simulink library "sm_trackV_lib_frame_idlerArm_i2u0l3"  (R2026a)
settings: Solver=VariableStepAuto
undefined symbols (not defined in the file): Trac, X, Y, Z
libraries: sm_lib x16
Description:
  | Copyright 2023-2026 The MathWorks, Inc.
settings Model: Creator=smiller  LastModifiedBy=smiller

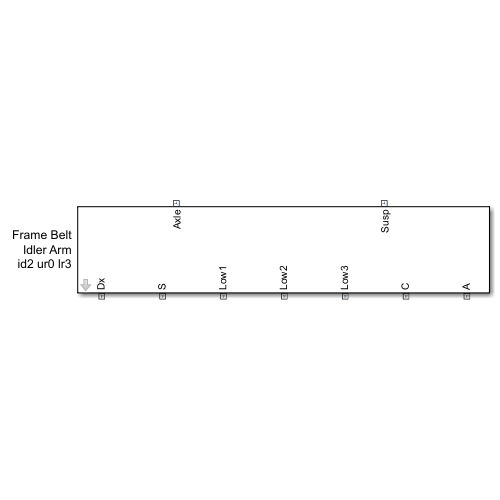
[thumbnail: Simulink's stored preview of the top-level diagram]
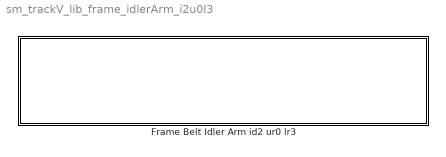
== system sm_trackV_lib_frame_idlerArm_i2u0l3 ==
  Frame Belt Idler Arm id2 ur0 lr3 : Subsystem  mask(Frame for Sprocket, Rollers (3), Fixed Idler, Idler Arm){popup_leftOrRight=Right, popup_trackFrame=Revolute, roller_lower_x=Trac.Frame.SprkOffLon.Lower, idlerArm_x=Trac.Frame.SprkOffLon.IdlerArm, idlerFix_x=Trac.Frame.SprkOffLon.IdlerR, tensionC_x=Trac.Frame.SprkOffLon.TensionC, frame_pivot_x=Trac.Frame.SprkOffLon.PivotFra, axle_x=Trac.Frame.SprkOffLon.Axle, roller_lower_y=Trac.Frame.SprkOffVer.Lower, idlerArm_y=Trac.Frame.SprkOffVer.IdlerArm, idlerFix_y=Trac.Frame.SprkOffVer.IdlerR, tensionC_y=Trac.Frame.SprkOffVer.TensionC, frame_pivot_y=Trac.Frame.SprkOffVer.PivotFra, axle_y=Trac.Frame.SprkOffVer.Axle, frame_roller_cg_offset=Trac.Frame.TrackFrame.CG, frame_roller_mass=Trac.Frame.TrackFrame.Mass, frame_roller_moi=Trac.Frame.TrackFrame.MOI, frame_roller_poi=Trac.Frame.TrackFrame.POI, frame_cg_offset=Trac.Frame.SprkFrame.CG, frame_mass=Trac.Frame.SprkFrame.Mass, frame_moi=Trac.Frame.SprkFrame.MOI, frame_poi=Trac.Frame.SprkFrame.POI, frame_susp_offset=Trac.Frame.SuspOffset, roller_frame_pivot_range=Trac.Frame.PivotFra.Range, roller_frame_pivot_k=Trac.Frame.PivotFra.LimitK, roller_frame_pivot_b=Trac.Frame.PivotFra.LimitB, roller_frame_pivot_tw=Trac.Frame.PivotFra.LimitTW}
      mask prompts: popup_leftOrRight "Left or Right"; popup_trackFrame "Track Frame"; roller_lower_x "Lower Rollers (vector) (m)"; idlerArm_x "Idler Arm (m)"; idlerFix_x "Idler Wheel Fixed (m)"; tensionC_x "Tensioner Cylinder (m)"; frame_pivot_x "Frame Pivot (m)"; axle_x "Axle (m)"; roller_lower_y "Lower Rollers (m)"; idlerArm_y "Idler Arm (m)"; idlerFix_y "Idler Wheel Fixed (m)"; tensionC_y "Tensioner Cylinder (m)"; frame_pivot_y "Frame Pivot (m)"; axle_y "Axle (m)"; frame_roller_cg_offset "CG Offset from Sprocket [x y z] (m)"; frame_roller_mass "Mass (kg)"; frame_roller_moi "Moments of Inertia [Ixx Iyy Izz] (kg*m^2)"; frame_roller_poi "Products of Inertia [Ixx Iyy Izz] (kg*m^2)"; frame_cg_offset "CG Offset from Sprocket [x y z] (m)"; frame_mass "Mass (kg)"; frame_moi "Moments of Inertia [Ixx Iyy Izz] (kg*m^2)"; frame_poi "Products of Inertia [Ixx Iyy Izz] (kg*m^2)"; frame_susp_offset "Suspension Offset from Sprocket [x y z] (m)"; roller_frame_pivot_range "Range (deg)"; roller_frame_pivot_k "Stop stiffness (N*m/deg)"; roller_frame_pivot_b "Stop damping (N*m/(deg*sec)"; roller_frame_pivot_tw "Stop transition width (deg)"
      mask help: Models frame locations for sprocket, 3 lower rollers, 1 fixed idler, 1 idler arm, and tensioner cylinder. Frame positions are all relative to sprocket center.
      mask init:
      | set_param([gcb '/Frame Connection'],'LabelModeActiveChoice',...
      |     get_param(gcb,'popup_trackFrame'))
      mask TypeOptions popup_trackFrame: Revolute | Fixed
      mask TypeOptions roller_frame_pivot_range: Frame Connection/roller_frame_pivot_range
      mask TypeOptions roller_frame_pivot_k: Frame Connection/roller_frame_pivot_k
      mask TypeOptions roller_frame_pivot_b: Frame Connection/roller_frame_pivot_b
      mask TypeOptions roller_frame_pivot_tw: Frame Connection/roller_frame_pivot_tw
      mask DialogControl cont_frame Prompt: Frame
      mask DialogControl cont_offset_x Prompt: Longitudinal Offsets from Sprocket
      mask DialogControl cont_offset_y Prompt: Vertical Offsets
      mask DialogControl cont_mass Prompt: Mass and Inertia
      mask DialogControl cont_roller_frame Prompt: Roller Frame
      mask DialogControl cont_sprk_frame Prompt: Sprocket_frame
      mask DialogControl cont_susp Prompt: Suspension Offsets
      mask DialogControl cont_framepviot Prompt: Frame Pivot (revolute only)

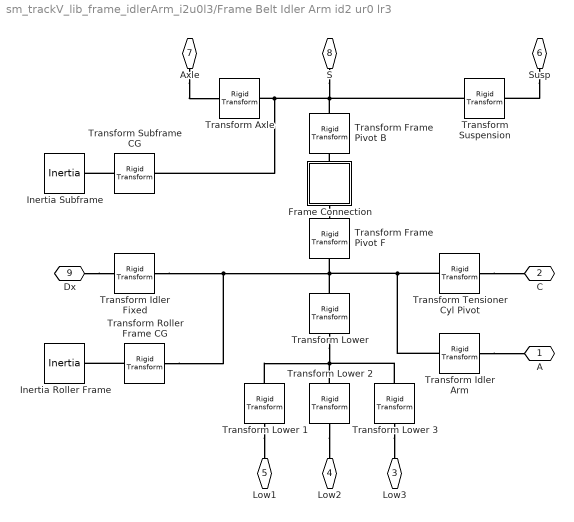
== system sm_trackV_lib_frame_idlerArm_i2u0l3/Frame Belt Idler Arm id2 ur0 lr3 ==
  Frame Connection : Subsystem  Variant=on  VariantControlMode=label  VariantControl=Revolute  LabelModeActiveChoice=Revolute  mask{roller_frame_pivot_range=roller_frame_pivot_range, roller_frame_pivot_k=roller_frame_pivot_k, roller_frame_pivot_b=roller_frame_pivot_b, roller_frame_pivot_tw=roller_frame_pivot_tw}
      mask prompts: roller_frame_pivot_range "Roller frame pivot range (deg)"; roller_frame_pivot_k "Roller frame pivot stop stiffness (N*m/deg)"; roller_frame_pivot_b "Roller frame pivot stop damping(N*m/(deg*sec)"; roller_frame_pivot_tw "Roller frame pivot stop transition width (deg)"
      settings: AttributesFormatString=%<LabelModeActiveChoice>
      mask Display: disp(' ')
  Inertia Roller Frame : sm_lib/Body Elements/Inertia  InertiaType=Custom  Mass=frame_roller_mass  MassUnits=kg  CenterOfMass=[0 0 0]  CenterOfMassUnits=m  MomentsOfInertia=frame_roller_moi  MomentsOfInertiaUnits=kg*m^2  ProductsOfInertia=frame_roller_poi  ProductsOfInertiaUnits=kg*m^2  GraphicType=None  MarkerShape=Frame  MarkerSize=20  GraphicVisPropType=SimpleVisualProperties  GraphicDiffuseColor=[0.5 0.5 0.5]  GraphicOpacity=1.0  GraphicSpecularColor=[0.5 0.5 0.5 1.0]  GraphicAmbientColor=[0.15 0.15 0.15 1.0]  GraphicEmissiveColor=[0.0 0.0 0.0 1.0]  GraphicShininess=75
  "Inertia Subframe " : sm_lib/Body Elements/Inertia  InertiaType=Custom  Mass=frame_mass  MassUnits=kg  CenterOfMass=[0 0 0]  CenterOfMassUnits=m  MomentsOfInertia=frame_moi  MomentsOfInertiaUnits=kg*m^2  ProductsOfInertia=frame_poi  ProductsOfInertiaUnits=kg*m^2  GraphicType=None  MarkerShape=Frame  MarkerSize=20  GraphicVisPropType=SimpleVisualProperties  GraphicDiffuseColor=[0.5 0.5 0.5]  GraphicOpacity=1.0  GraphicSpecularColor=[0.5 0.5 0.5 1.0]  GraphicAmbientColor=[0.15 0.15 0.15 1.0]  GraphicEmissiveColor=[0.0 0.0 0.0 1.0]  GraphicShininess=75
  Transform Axle : sm_lib/Frames and Transforms/Rigid Transform  RotationMethod=None  FollAlignAxisA=+X  BaseAlignAxisA=+Y  FollAlignAxisB=+Y  BaseAlignAxisB=+Z  RotationStandardAxis=+Z  RotationAngle=0.0  RotationAngleUnits=deg  RotationArbitraryAxis=[0 0 1]  RotationSequenceAxes=FollowerAxes  RotationSequence=XYX  RotationSequenceAngles=[0 0 0]  RotationSequenceAnglesUnits=deg  RotationMatrix=[1 0 0; 0 1 0; 0 0 1]  Quaternion=[1 0 0 0]  TranslationMethod=Cartesian  TranslationCartesianOffset=[axle_x -axle_y 0]  TranslationCartesianOffsetUnits=m  TranslationStandardAxis=+X  TranslationStandardOffset=0  TranslationStandardOffsetUnits=m  TranslationROffset=0  TranslationROffsetUnits=m  TranslationThetaOffset=0  TranslationThetaOffsetUnits=deg  TranslationZOffset=0  TranslationZOffsetUnits=m
  Transform Frame Pivot B : sm_lib/Frames and Transforms/Rigid Transform  RotationMethod=None  FollAlignAxisA=+X  BaseAlignAxisA=+Y  FollAlignAxisB=+Y  BaseAlignAxisB=+Z  RotationStandardAxis=+Z  RotationAngle=0.0  RotationAngleUnits=deg  RotationArbitraryAxis=[0 0 1]  RotationSequenceAxes=FollowerAxes  RotationSequence=XYX  RotationSequenceAngles=[0 0 0]  RotationSequenceAnglesUnits=deg  RotationMatrix=[1 0 0; 0 1 0; 0 0 1]  Quaternion=[1 0 0 0]  TranslationMethod=Cartesian  TranslationCartesianOffset=[frame_pivot_x -frame_pivot_y 0]  TranslationCartesianOffsetUnits=m  TranslationStandardAxis=+Z  TranslationStandardOffset=0  TranslationStandardOffsetUnits=m  TranslationROffset=0  TranslationROffsetUnits=m  TranslationThetaOffset=0  TranslationThetaOffsetUnits=deg  TranslationZOffset=0  TranslationZOffsetUnits=m
  Transform Frame Pivot F : sm_lib/Frames and Transforms/Rigid Transform  RotationMethod=None  FollAlignAxisA=+X  BaseAlignAxisA=+Y  FollAlignAxisB=+Y  BaseAlignAxisB=+Z  RotationStandardAxis=+Z  RotationAngle=0.0  RotationAngleUnits=deg  RotationArbitraryAxis=[0 0 1]  RotationSequenceAxes=FollowerAxes  RotationSequence=XYX  RotationSequenceAngles=[0 0 0]  RotationSequenceAnglesUnits=deg  RotationMatrix=[1 0 0; 0 1 0; 0 0 1]  Quaternion=[1 0 0 0]  TranslationMethod=Cartesian  TranslationCartesianOffset=[frame_pivot_x -frame_pivot_y 0]  TranslationCartesianOffsetUnits=m  TranslationStandardAxis=+Z  TranslationStandardOffset=0  TranslationStandardOffsetUnits=m  TranslationROffset=0  TranslationROffsetUnits=m  TranslationThetaOffset=0  TranslationThetaOffsetUnits=deg  TranslationZOffset=0  TranslationZOffsetUnits=m
  Transform Idler Arm : sm_lib/Frames and Transforms/Rigid Transform  RotationMethod=None  FollAlignAxisA=+X  BaseAlignAxisA=+Y  FollAlignAxisB=+Y  BaseAlignAxisB=+Z  RotationStandardAxis=+Z  RotationAngle=0.0  RotationAngleUnits=deg  RotationArbitraryAxis=[0 0 1]  RotationSequenceAxes=FollowerAxes  RotationSequence=XYX  RotationSequenceAngles=[0 0 0]  RotationSequenceAnglesUnits=deg  RotationMatrix=[1 0 0; 0 1 0; 0 0 1]  Quaternion=[1 0 0 0]  TranslationMethod=Cartesian  TranslationCartesianOffset=[idlerArm_x -idlerArm_y 0]  TranslationCartesianOffsetUnits=m  TranslationStandardAxis=+Z  TranslationStandardOffset=0  TranslationStandardOffsetUnits=m  TranslationROffset=0  TranslationROffsetUnits=m  TranslationThetaOffset=0  TranslationThetaOffsetUnits=deg  TranslationZOffset=0  TranslationZOffsetUnits=m
  Transform Idler Fixed : sm_lib/Frames and Transforms/Rigid Transform  RotationMethod=None  FollAlignAxisA=+X  BaseAlignAxisA=+Y  FollAlignAxisB=+Y  BaseAlignAxisB=+Z  RotationStandardAxis=+Z  RotationAngle=0.0  RotationAngleUnits=deg  RotationArbitraryAxis=[0 0 1]  RotationSequenceAxes=FollowerAxes  RotationSequence=XYX  RotationSequenceAngles=[0 0 0]  RotationSequenceAnglesUnits=deg  RotationMatrix=[1 0 0; 0 1 0; 0 0 1]  Quaternion=[1 0 0 0]  TranslationMethod=Cartesian  TranslationCartesianOffset=[idlerFix_x -idlerFix_y 0]  TranslationCartesianOffsetUnits=m  TranslationStandardAxis=+Z  TranslationStandardOffset=0  TranslationStandardOffsetUnits=m  TranslationROffset=0  TranslationROffsetUnits=m  TranslationThetaOffset=0  TranslationThetaOffsetUnits=deg  TranslationZOffset=0  TranslationZOffsetUnits=m
  Transform Lower : sm_lib/Frames and Transforms/Rigid Transform  RotationMethod=None  FollAlignAxisA=+X  BaseAlignAxisA=+Y  FollAlignAxisB=+Y  BaseAlignAxisB=+Z  RotationStandardAxis=+X  RotationAngle=90  RotationAngleUnits=deg  RotationArbitraryAxis=[0 0 1]  RotationSequenceAxes=FollowerAxes  RotationSequence=XYX  RotationSequenceAngles=[0 0 0]  RotationSequenceAnglesUnits=deg  RotationMatrix=[1 0 0; 0 1 0; 0 0 1]  Quaternion=[1 0 0 0]  TranslationMethod=StandardAxis  TranslationCartesianOffset=[-46.4567 43.3071 -1.4567]  TranslationCartesianOffsetUnits=m  TranslationStandardAxis=+Y  TranslationStandardOffset=-roller_lower_y  TranslationStandardOffsetUnits=m  TranslationROffset=0  TranslationROffsetUnits=m  TranslationThetaOffset=0  TranslationThetaOffsetUnits=deg  TranslationZOffset=0  TranslationZOffsetUnits=m
  Transform Lower 1 : sm_lib/Frames and Transforms/Rigid Transform  RotationMethod=None  FollAlignAxisA=+X  BaseAlignAxisA=+Y  FollAlignAxisB=+Y  BaseAlignAxisB=+Z  RotationStandardAxis=+Z  RotationAngle=0.0  RotationAngleUnits=deg  RotationArbitraryAxis=[0 0 1]  RotationSequenceAxes=FollowerAxes  RotationSequence=XYX  RotationSequenceAngles=[0 0 0]  RotationSequenceAnglesUnits=deg  RotationMatrix=[1 0 0; 0 1 0; 0 0 1]  Quaternion=[1 0 0 0]  TranslationMethod=StandardAxis  TranslationCartesianOffset=[0 0 0]  TranslationCartesianOffsetUnits=m  TranslationStandardAxis=+X  TranslationStandardOffset=roller_lower_x(1)  TranslationStandardOffsetUnits=m  TranslationROffset=0  TranslationROffsetUnits=m  TranslationThetaOffset=0  TranslationThetaOffsetUnits=deg  TranslationZOffset=0  TranslationZOffsetUnits=m
  Transform Lower 2 : sm_lib/Frames and Transforms/Rigid Transform  RotationMethod=None  FollAlignAxisA=+X  BaseAlignAxisA=+Y  FollAlignAxisB=+Y  BaseAlignAxisB=+Z  RotationStandardAxis=+Z  RotationAngle=0.0  RotationAngleUnits=deg  RotationArbitraryAxis=[0 0 1]  RotationSequenceAxes=FollowerAxes  RotationSequence=XYX  RotationSequenceAngles=[0 0 0]  RotationSequenceAnglesUnits=deg  RotationMatrix=[1 0 0; 0 1 0; 0 0 1]  Quaternion=[1 0 0 0]  TranslationMethod=StandardAxis  TranslationCartesianOffset=[0 0 0]  TranslationCartesianOffsetUnits=m  TranslationStandardAxis=+X  TranslationStandardOffset=roller_lower_x(2)  TranslationStandardOffsetUnits=m  TranslationROffset=0  TranslationROffsetUnits=m  TranslationThetaOffset=0  TranslationThetaOffsetUnits=deg  TranslationZOffset=0  TranslationZOffsetUnits=m
  Transform Lower 3 : sm_lib/Frames and Transforms/Rigid Transform  RotationMethod=None  FollAlignAxisA=+X  BaseAlignAxisA=+Y  FollAlignAxisB=+Y  BaseAlignAxisB=+Z  RotationStandardAxis=+Z  RotationAngle=0.0  RotationAngleUnits=deg  RotationArbitraryAxis=[0 0 1]  RotationSequenceAxes=FollowerAxes  RotationSequence=XYX  RotationSequenceAngles=[0 0 0]  RotationSequenceAnglesUnits=deg  RotationMatrix=[1 0 0; 0 1 0; 0 0 1]  Quaternion=[1 0 0 0]  TranslationMethod=StandardAxis  TranslationCartesianOffset=[0 0 0]  TranslationCartesianOffsetUnits=m  TranslationStandardAxis=+X  TranslationStandardOffset=roller_lower_x(3)  TranslationStandardOffsetUnits=m  TranslationROffset=0  TranslationROffsetUnits=m  TranslationThetaOffset=0  TranslationThetaOffsetUnits=deg  TranslationZOffset=0  TranslationZOffsetUnits=m
  Transform Roller Frame CG : sm_lib/Frames and Transforms/Rigid Transform  RotationMethod=None  FollAlignAxisA=+X  BaseAlignAxisA=+Y  FollAlignAxisB=+Y  BaseAlignAxisB=+Z  RotationStandardAxis=+Z  RotationAngle=0.0  RotationAngleUnits=deg  RotationArbitraryAxis=[0 0 1]  RotationSequenceAxes=FollowerAxes  RotationSequence=XYX  RotationSequenceAngles=[0 0 0]  RotationSequenceAnglesUnits=deg  RotationMatrix=[1 0 0; 0 1 0; 0 0 1]  Quaternion=[1 0 0 0]  TranslationMethod=Cartesian  TranslationCartesianOffset=frame_cg_offset.*[1 -1 1]  TranslationCartesianOffsetUnits=m  TranslationStandardAxis=+Z  TranslationStandardOffset=0  TranslationStandardOffsetUnits=m  TranslationROffset=0  TranslationROffsetUnits=m  TranslationThetaOffset=0  TranslationThetaOffsetUnits=deg  TranslationZOffset=0  TranslationZOffsetUnits=m
  Transform Subframe CG : sm_lib/Frames and Transforms/Rigid Transform  RotationMethod=None  FollAlignAxisA=+X  BaseAlignAxisA=+Y  FollAlignAxisB=+Y  BaseAlignAxisB=+Z  RotationStandardAxis=+Z  RotationAngle=0.0  RotationAngleUnits=deg  RotationArbitraryAxis=[0 0 1]  RotationSequenceAxes=FollowerAxes  RotationSequence=XYX  RotationSequenceAngles=[0 0 0]  RotationSequenceAnglesUnits=deg  RotationMatrix=[1 0 0; 0 1 0; 0 0 1]  Quaternion=[1 0 0 0]  TranslationMethod=Cartesian  TranslationCartesianOffset=frame_cg_offset.*[1 -1 1]  TranslationCartesianOffsetUnits=m  TranslationStandardAxis=+Z  TranslationStandardOffset=0  TranslationStandardOffsetUnits=m  TranslationROffset=0  TranslationROffsetUnits=m  TranslationThetaOffset=0  TranslationThetaOffsetUnits=deg  TranslationZOffset=0  TranslationZOffsetUnits=m
  Transform Suspension : sm_lib/Frames and Transforms/Rigid Transform  RotationMethod=None  FollAlignAxisA=+X  BaseAlignAxisA=+Y  FollAlignAxisB=+Y  BaseAlignAxisB=+Z  RotationStandardAxis=+Z  RotationAngle=0.0  RotationAngleUnits=deg  RotationArbitraryAxis=[0 0 1]  RotationSequenceAxes=FollowerAxes  RotationSequence=XYX  RotationSequenceAngles=[0 0 0]  RotationSequenceAnglesUnits=deg  RotationMatrix=[1 0 0; 0 1 0; 0 0 1]  Quaternion=[1 0 0 0]  TranslationMethod=Cartesian  TranslationCartesianOffset=frame_susp_offset.*[1 -1 popup_leftOrRight ]  TranslationCartesianOffsetUnits=m  TranslationStandardAxis=+Z  TranslationStandardOffset=0  TranslationStandardOffsetUnits=m  TranslationROffset=0  TranslationROffsetUnits=m  TranslationThetaOffset=0  TranslationThetaOffsetUnits=deg  TranslationZOffset=0  TranslationZOffsetUnits=m
  Transform Tensioner Cyl Pivot : sm_lib/Frames and Transforms/Rigid Transform  RotationMethod=None  FollAlignAxisA=+Z  BaseAlignAxisA=+X  FollAlignAxisB=+X  BaseAlignAxisB=+Y  RotationStandardAxis=+Y  RotationAngle=90  RotationAngleUnits=deg  RotationArbitraryAxis=[0 0 1]  RotationSequenceAxes=FollowerAxes  RotationSequence=XYX  RotationSequenceAngles=[0 0 0]  RotationSequenceAnglesUnits=deg  RotationMatrix=[1 0 0; 0 1 0; 0 0 1]  Quaternion=[1 0 0 0]  TranslationMethod=Cartesian  TranslationCartesianOffset=[tensionC_x -tensionC_y 0]  TranslationCartesianOffsetUnits=m  TranslationStandardAxis=+Z  TranslationStandardOffset=0  TranslationStandardOffsetUnits=m  TranslationROffset=0  TranslationROffsetUnits=m  TranslationThetaOffset=0  TranslationThetaOffsetUnits=deg  TranslationZOffset=0  TranslationZOffsetUnits=m
  A : PMIOPort  Side=Right
  C : PMIOPort  Port=2  Side=Right
  Low3 : PMIOPort  Port=3  Side=Right
  Low2 : PMIOPort  Port=4  Side=Right
  Low1 : PMIOPort  Port=5  Side=Right
  Susp : PMIOPort  Port=6  Side=Left
  Axle : PMIOPort  Port=7  Side=Left
  S : PMIOPort  Port=8  Side=Right
  Dx : PMIOPort  Port=9  Side=Right
  connections:
  Transform Lower 3/RConn1 -- Low3/RConn1
  Transform Tensioner Cyl Pivot/RConn1 -- C/RConn1
  Transform Roller Frame CG/RConn1 -- Inertia Roller Frame/RConn1
  Transform Idler Arm/RConn1 -- A/RConn1
  Transform Frame Pivot F/LConn1 -- Transform Tensioner Cyl Pivot/LConn1 -- Transform Idler Arm/LConn1 -- Transform Idler Fixed/LConn1 -- Transform Roller Frame CG/LConn1 -- Transform Lower/LConn1
  Dx/RConn1 -- Transform Idler Fixed/RConn1
  Transform Lower 2/RConn1 -- Low2/RConn1
  Transform Axle/LConn1 -- Transform Suspension/LConn1 -- Transform Frame Pivot B/LConn1 -- S/RConn1 -- Transform Subframe CG/LConn1
  Transform Lower 1/RConn1 -- Low1/RConn1
  Transform Lower/RConn1 -- Transform Lower 2/LConn1 -- Transform Lower 3/LConn1 -- Transform Lower 1/LConn1
  Transform Subframe CG/RConn1 -- "Inertia Subframe "/RConn1
  Axle/RConn1 -- Transform Axle/RConn1
  Susp/RConn1 -- Transform Suspension/RConn1
  Frame Connection/LConn1 -- Transform Frame Pivot B/RConn1
  Frame Connection/RConn1 -- Transform Frame Pivot F/RConn1

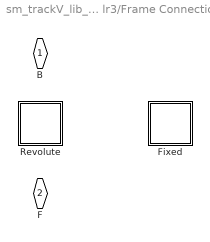
== system sm_trackV_lib_frame_idlerArm_i2u0l3/Frame Belt Idler Arm id2 ur0 lr3/Frame Connection ==
  Fixed : Subsystem  VariantControl=Fixed
  Revolute : Subsystem  VariantControl=Revolute
  B : PMIOPort  Side=Left
  F : PMIOPort  Port=2  Side=Right

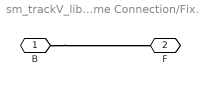
== system sm_trackV_lib_frame_idlerArm_i2u0l3/Frame Belt Idler Arm id2 ur0 lr3/Frame Connection/Fixed ==
  B : PMIOPort  Side=Left
  F : PMIOPort  Port=2  Side=Right
  connections:
  B/RConn1 -- F/RConn1

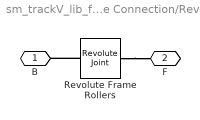
== system sm_trackV_lib_frame_idlerArm_i2u0l3/Frame Belt Idler Arm id2 ur0 lr3/Frame Connection/Revolute ==
  Revolute Frame Rollers : sm_lib/Joints/Revolute Joint  JointMode=Normal  CompositeWrenchDir=FollowerOnBase  CompositeWrenchFrame=BaseFrame  SenseConstraintForce=off  SenseConstraintTorque=off  SenseTotalForce=off  SenseTotalTorque=off  PositionTargetSpecify=on  PositionTargetPriority=High  PositionTargetValue=0  PositionTargetValueUnits=deg  VelocityTargetSpecify=off  VelocityTargetPriority=High  VelocityTargetValue=0  VelocityTargetValueUnits=deg/s  EquilibriumPosition=0  EquilibriumPositionUnits=deg  SpringStiffness=0  SpringStiffnessUnits=N*m/deg  DampingCoefficient=0  DampingCoefficientUnits=N*m/(deg/s)  LowerLimitSpecify=on  LowerLimitBound=-roller_frame_pivot_range/2  LowerLimitBoundUnits=deg  LowerLimitStiffness=roller_frame_pivot_k  LowerLimitStiffnessUnits=N*m/deg  LowerLimitDamping=roller_frame_pivot_b  LowerLimitDampingUnits=N*m/(deg/s)  LowerLimitTransitionRegionWidth=roller_frame_pivot_tw  LowerLimitTransitionRegionWidthUnits=deg  UpperLimitSpecify=on  UpperLimitBound=roller_frame_pivot_range/2  UpperLimitBoundUnits=deg  UpperLimitStiffness=roller_frame_pivot_k  UpperLimitStiffnessUnits=N*m/deg  UpperLimitDamping=roller_frame_pivot_b  UpperLimitDampingUnits=N*m/(deg/s)  UpperLimitTransitionRegionWidth=roller_frame_pivot_tw  UpperLimitTransitionRegionWidthUnits=deg  TorqueActuationMode=NoTorque  MotionActuationMode=ComputedMotion  SensePosition=off  SenseVelocity=off  SenseAcceleration=off  SenseTorqueForce=off  SenseLowerLimitTorqueForce=off  SenseUpperLimitTorqueForce=off
  B : PMIOPort  Side=Left
  F : PMIOPort  Port=2  Side=Right
  connections:
  Revolute Frame Rollers/RConn1 -- F/RConn1
  Revolute Frame Rollers/LConn1 -- B/RConn1
